simulink model "posmall_2016"  (R2016b)
settings: Solver=ode23tb  StartTime=0.0  StopTime=0.6  RelTol=1e-3
libraries: powerlib x19, re_lib x2, powerlib_meascontrol x2
settings Model: Creator=Muhi zatar  LastModifiedBy=Muhi zatar
settings SimscapeCC: SimscapeNormalizeSystem=off

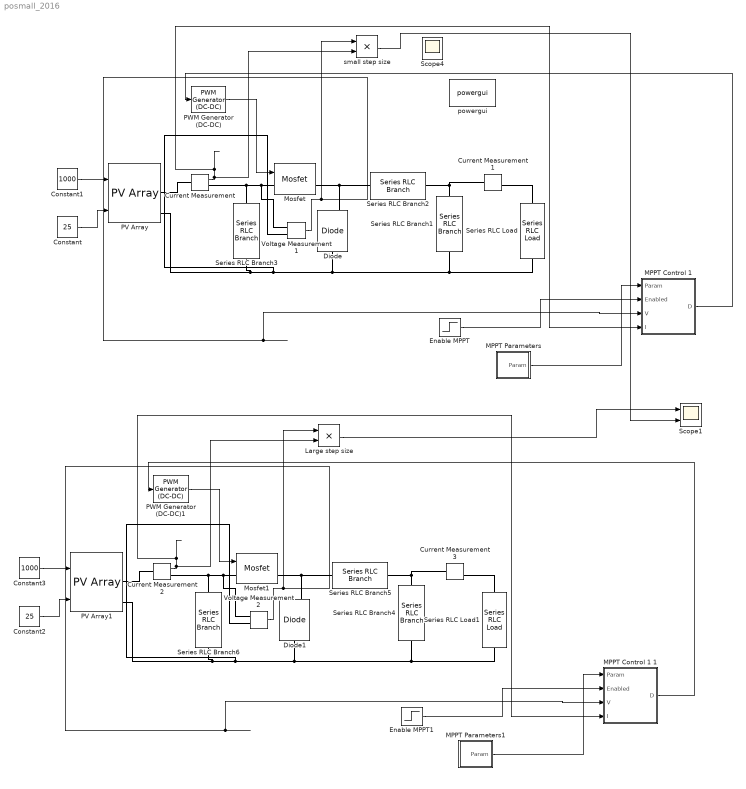
== system posmall_2016 ==
  Constant : Constant  Value=25
  Constant1 : Constant  Value=1000
  Constant2 : Constant  Value=25
  Constant3 : Constant  Value=1000
  Current Measurement{,1..3} (4 alike) : powerlib/Measurements/Current Measurement  PhasorSimulation=off  OutputType=Complex  PSBequivalent=0
  Diode : powerlib/Power Electronics/Diode  Ron=0.000001  Lon=0  Vf=0  IC=0  UseSnubber=off  Rs=500  Cs=250e-9  Measurements=on
  Diode1 : powerlib/Power Electronics/Diode  Ron=0.000001  Lon=0  Vf=0  IC=0  UseSnubber=off  Rs=500  Cs=250e-9  Measurements=on
  Enable MPPT : Step  Time=0  SampleTime=0
  Enable MPPT1 : Step  Time=0  SampleTime=0
  Large step size : Product
  MPPT Parameters : Subsystem
  MPPT Parameters1 : Subsystem
  "MPPT Control 1 " : MATLAB Function  TreatAsAtomicUnit=on
  MPPT Control 1 1 : MATLAB Function  TreatAsAtomicUnit=on
  Mosfet : powerlib/Power Electronics/Mosfet  Ron=0.0000001  Lon=0  Rd=0.0000001  Vfd=0  IC=0  Rs=1e5  Cs=inf  Measurements=on
  Mosfet1 : powerlib/Power Electronics/Mosfet  Ron=0.0000001  Lon=0  Rd=0.0000001  Vfd=0  IC=0  Rs=1e5  Cs=inf  Measurements=on
  PV Array : re_lib/Solar/PV Array  Npar=1  Nser=1  PlotType=array @ 25 deg.C & specified irradiances  S_vec="[ 1000  800  500 ]"  Temp_C_vec="[ 45 25  ]"  ModuleName=1Soltech 1STH-215-P  PlotWhenSelected=off  Pm=213.15  Ncell=60  Voc=36.3  Isc=7.84  Vm=29  Im=7.35  beta_Voc_pc=-0.36099  alpha_Isc_pc=0.102  beta_Voc=-0.13104  alpha_Isc=0.007997  IL=7.8649  I0=2.9259e-10  nI=0.98117  Rsh=313.3991  Rs=0.39383  BAL=off  Tc=1e-6  Tfilter=5e-5
  PV Array1 : re_lib/Solar/PV Array  Npar=1  Nser=1  PlotType=array @ 25 deg.C & specified irradiances  S_vec="[ 1000  800  500 ]"  Temp_C_vec="[ 45 25  ]"  ModuleName=1Soltech 1STH-215-P  PlotWhenSelected=off  Pm=213.15  Ncell=60  Voc=36.3  Isc=7.84  Vm=29  Im=7.35  beta_Voc_pc=-0.36099  alpha_Isc_pc=0.102  beta_Voc=-0.13104  alpha_Isc=0.007997  IL=7.8649  I0=2.9259e-10  nI=0.98117  Rsh=313.3991  Rs=0.39383  BAL=off  Tc=1e-6  Tfilter=5e-5
  PWM Generator (DC-DC) : powerlib_meascontrol/Pulse & Signal Generators/PWM Generator (DC-DC)  Fsw=50000  Ts=0
  PWM Generator (DC-DC)1 : powerlib_meascontrol/Pulse & Signal Generators/PWM Generator (DC-DC)  Fsw=50000  Ts=0
  Scope1 : Scope  NumInputPorts=2
  Scope4 : Scope
  Series RLC Branch1 : powerlib/Elements/Series RLC Branch  LConnTagsString=__new0  RConnTagsString=__new0  BranchType=C  Resistance=0.01  Inductance=1e-3  SetiL0=off  InitialCurrent=0  Capacitance=1e-3  Setx0=off  InitialVoltage=0  Measurements=None
  Series RLC Branch2 : powerlib/Elements/Series RLC Branch  LConnTagsString=__new0  RConnTagsString=__new0  BranchType=L  Resistance=5  Inductance=1e-3  SetiL0=off  InitialCurrent=0  Capacitance=1e-6  Setx0=off  InitialVoltage=0  Measurements=None
  Series RLC Branch3 : powerlib/Elements/Series RLC Branch  LConnTagsString=__new0  RConnTagsString=__new0  BranchType=C  Resistance=5  Inductance=1e-3  SetiL0=off  InitialCurrent=0  Capacitance=1e-3  Setx0=off  InitialVoltage=0  Measurements=None
  Series RLC Branch4 : powerlib/Elements/Series RLC Branch  LConnTagsString=__new0  RConnTagsString=__new0  BranchType=C  Resistance=0.01  Inductance=1e-3  SetiL0=off  InitialCurrent=0  Capacitance=1e-3  Setx0=off  InitialVoltage=0  Measurements=None
  Series RLC Branch5 : powerlib/Elements/Series RLC Branch  LConnTagsString=__new0  RConnTagsString=__new0  BranchType=L  Resistance=5  Inductance=1e-3  SetiL0=off  InitialCurrent=0  Capacitance=1e-6  Setx0=off  InitialVoltage=0  Measurements=None
  Series RLC Branch6 : powerlib/Elements/Series RLC Branch  LConnTagsString=__new0  RConnTagsString=__new0  BranchType=C  Resistance=5  Inductance=1e-3  SetiL0=off  InitialCurrent=0  Capacitance=1e-3  Setx0=off  InitialVoltage=0  Measurements=None
  Series RLC Load : powerlib/Elements/Series RLC Load  LConnTagsString=a  RConnTagsString=__new0  NominalVoltage=15  NominalFrequency=60  ActivePower=210  InductivePower=0  CapacitivePower=0  Setx0=off  InitialVoltage=0  SetiL0=off  InitialCurrent=0  Measurements=None  LoadType=constant Z
  Series RLC Load1 : powerlib/Elements/Series RLC Load  LConnTagsString=a  RConnTagsString=__new0  NominalVoltage=15  NominalFrequency=60  ActivePower=210  InductivePower=0  CapacitivePower=0  Setx0=off  InitialVoltage=0  SetiL0=off  InitialCurrent=0  Measurements=None  LoadType=constant Z
  Voltage Measurement1 : powerlib/Measurements/Voltage Measurement  PhasorSimulation=off  OutputType=Complex  PSBequivalent=0
  Voltage Measurement2 : powerlib/Measurements/Voltage Measurement  PhasorSimulation=off  OutputType=Complex  PSBequivalent=0
  powergui : powerlib/powergui  Priority=1  SimulationMode=Discrete  SampleTime=1e-7  frequency=60  Iterations=50  frequencyindice=0  Pbase=100e6  ErrMax=1e-4  UnitsV=kV  UnitsW=MW  buscounter=0  FunctionMessages=off  echomessages=off  EnableUseOfTLC=off  CurrentSourceSwitches=off  DisableSnubberDevices=off  DisableRonSwitches=off  DisableVfSwitches=off  DisplayEquations=off  SolverType=Tustin/Backward Euler (TBE)  Interpol=off  ExternalGateDelay=off  methode=off  Ts=10  x0status=blocks  SPID=off  SwTol=0  HookPort=off  RestoreLinks=warning  ResistiveCurrentMeasurement=off  Frange=[0:2:500]  Ylog=off  Xlog=on  ShowGrid=off  save=off  variable=ZData  structure=0  ZoomFFT=off  StartTime=0.0  cycles=1  DisplayStyle=1  fundamental=60  FreqAxis=off  MaxFrequency=1000  frequencyindicesteady=1  RmsSteady=1  display=off
  small step size : Product
  wires:
  Constant/1 -> PV Array/2
  Current Measurement/1 -> small step size/2, "MPPT Control 1 "/4(I)
  PWM Generator (DC-DC)/1 -> Mosfet/1
  Voltage Measurement1/1 -> small step size/1, "MPPT Control 1 "/3(V)
  MPPT Parameters/1(Param) -> "MPPT Control 1 "/1(Param)
  Enable MPPT/1 -> "MPPT Control 1 "/2(Enabled)
  "MPPT Control 1 "/1(D) -> PWM Generator (DC-DC)/1
  Constant1/1 -> PV Array/1
  Constant2/1 -> PV Array1/2
  Current Measurement2/1 -> Large step size/2, MPPT Control 1 1/4(I)
  PWM Generator (DC-DC)1/1 -> Mosfet1/1
  Voltage Measurement2/1 -> Large step size/1, MPPT Control 1 1/3(V)
  Large step size/1 -> Scope1/1
  MPPT Parameters1/1(Param) -> MPPT Control 1 1/1(Param)
  Enable MPPT1/1 -> MPPT Control 1 1/2(Enabled)
  MPPT Control 1 1/1(D) -> PWM Generator (DC-DC)1/1
  Constant3/1 -> PV Array1/1
  small step size/1 -> Scope1/2
  connections:
  Voltage Measurement1/LConn1 -- Mosfet/LConn1 -- Current Measurement/RConn1 -- Series RLC Branch3/LConn1
  Mosfet/RConn1 -- Series RLC Branch2/LConn1 -- Diode/RConn1
  Series RLC Branch1/RConn1 -- Series RLC Load/RConn1 -- Diode/LConn1 -- Voltage Measurement1/LConn2 -- PV Array/RConn2 -- Series RLC Branch3/RConn1
  Series RLC Branch2/RConn1 -- Current Measurement1/LConn1 -- Series RLC Branch1/LConn1
  Current Measurement1/RConn1 -- Series RLC Load/LConn1
  Current Measurement/LConn1 -- PV Array/RConn1
  Voltage Measurement2/LConn1 -- Mosfet1/LConn1 -- Current Measurement2/RConn1 -- Series RLC Branch6/LConn1
  Mosfet1/RConn1 -- Series RLC Branch5/LConn1 -- Diode1/RConn1
  Series RLC Branch4/RConn1 -- Series RLC Load1/RConn1 -- Diode1/LConn1 -- Voltage Measurement2/LConn2 -- PV Array1/RConn2 -- Series RLC Branch6/RConn1
  Series RLC Branch5/RConn1 -- Current Measurement3/LConn1 -- Series RLC Branch4/LConn1
  Current Measurement3/RConn1 -- Series RLC Load1/LConn1
  Current Measurement2/LConn1 -- PV Array1/RConn1

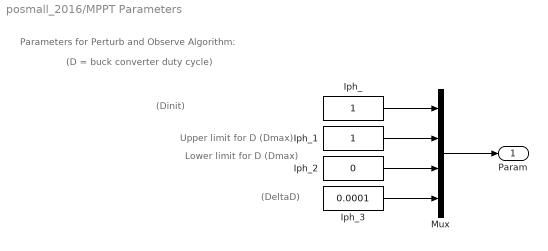
== system posmall_2016/MPPT Parameters ==
  note: Upper limit for D (Dmax)
  note: (DeltaD)
  note: (Dinit)
  note: (D = buck converter duty cycle)
  note: Lower limit for D (Dmax)
  note: Parameters for Perturb and Observe Algorithm:
  Iph_ : Constant
  Iph_1 : Constant
  Iph_2 : Constant  Value=0
  Iph_3 : Constant  Value=0.0001
  Mux : Mux
  Param : Outport
  wires:
  Iph_/1 -> Mux/1
  Iph_1/1 -> Mux/2
  Iph_2/1 -> Mux/3
  Iph_3/1 -> Mux/4
  Mux/1 -> Param/1

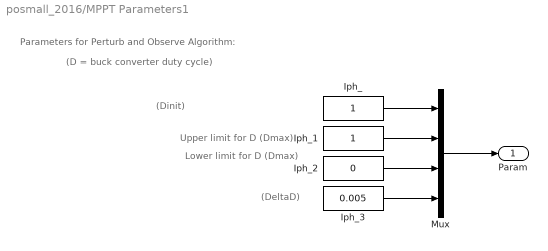
== system posmall_2016/MPPT Parameters1 ==
  note: Upper limit for D (Dmax)
  note: (DeltaD)
  note: (Dinit)
  note: (D = buck converter duty cycle)
  note: Lower limit for D (Dmax)
  note: Parameters for Perturb and Observe Algorithm:
  Iph_ : Constant
  Iph_1 : Constant
  Iph_2 : Constant  Value=0
  Iph_3 : Constant  Value=0.005
  Mux : Mux
  Param : Outport
  wires:
  Iph_/1 -> Mux/1
  Iph_1/1 -> Mux/2
  Iph_2/1 -> Mux/3
  Iph_3/1 -> Mux/4
  Mux/1 -> Param/1

== matlab function posmall_2016/MPPT Control 1 1 ==
  settings: updateMethod=DISCRETE  sampleTime=Ts_Control
  data: Param input; Enabled input; V input =V; I input; D output
function D  = PandO(Param, Enabled, V, I)

% MPPT controller based on the Perturb & Observe algorithm.

% D output = Duty cycle of the boost converter (value between 0 and 1)
%
% Enabled input = 1 to enable the MPPT controller
% V input = PV array terminal voltage (V)
% I input = PV array current (A)
%
% Param input:
Dinit = Param(1);  %Initial value for D output
Dmax = Param(2);   %Maximum value for D
Dmin = Param(3);   %Minimum value for D
deltaD = Param(4); %Increment value used to increase/decrease the duty cycle D
% ( increasing D = decreasing Vref )
%  

persistent Vold Pold Dold;

dataType = 'double';

if isempty(Vold)
    Vold=0;
    Pold=0;
    Dold=Dinit;
end
P= V*I;
dV= V - Vold;
dP= P - Pold;

if dP ~= 0 & Enabled ~=0
    if dP < 0
        if dV < 0
            D = Dold - deltaD;
        else
            D = Dold + deltaD;
        end
    else
        if dV < 0
            D = Dold + deltaD;
        else
            D = Dold - deltaD;
        end    
    end
else D=Dold;
end

if D >= Dmax | D<= Dmin
    D=Dold;
end

Dold=D;
Vold=V;
Pold=P;

== matlab function posmall_2016/MPPT Control 1  ==
  settings: updateMethod=DISCRETE  sampleTime=Ts_Control
  data: Param input; Enabled input; V input =V; I input; D output
function D  = PandO(Param, Enabled, V, I)

% MPPT controller based on the Perturb & Observe algorithm.

% D output = Duty cycle of the boost converter (value between 0 and 1)
%
% Enabled input = 1 to enable the MPPT controller
% V input = PV array terminal voltage (V)
% I input = PV array current (A)
%
% Param input:
Dinit = Param(1);  %Initial value for D output
Dmax = Param(2);   %Maximum value for D
Dmin = Param(3);   %Minimum value for D
deltaD = Param(4); %Increment value used to increase/decrease the duty cycle D
% ( increasing D = decreasing Vref )
%  

persistent Vold Pold Dold;

dataType = 'double';

if isempty(Vold)
    Vold=0;
    Pold=0;
    Dold=Dinit;
end
P= V*I;
dV= V - Vold;
dP= P - Pold;

if dP ~= 0 & Enabled ~=0
    if dP < 0
        if dV < 0
            D = Dold - deltaD;
        else
            D = Dold + deltaD;
        end
    else
        if dV < 0
            D = Dold + deltaD;
        else
            D = Dold - deltaD;
        end    
    end
else D=Dold;
end

if D >= Dmax | D<= Dmin
    D=Dold;
end

Dold=D;
Vold=V;
Pold=P;
